simulink model "LoFT_Example3"  (R2024b)
settings: Solver=ode4  StartTime=0.0  StopTime=300  FixedStep=simu.dt  RelTol=1e-3
undefined symbols (not defined in the file): body, circtime, Communication, D1, Delta, irkb, line, LoFT, p0, Pn, s, simu, trip_time, Turbwind, waves, wind
libraries: simulink x350, spsThreePhaseVIMeasurementLib x41, spsThreePhasePISectionLineLib x34, spsThreePhaseParallelRLCLoadLib x21, spsThreePhaseTransformerTwoWindingsLib x14, spsLoadFlowBusLib x10, spsThreePhaseDynamicLoadLib x9, spsSynchronousMachinepuStandardLib x7, spsExcitationSystemLib x7, spsSteamTurbineandGovernorLib x7, spsGenericPowerSystemStabilizerLib x7, spsMultiBandPowerSystemStabilizerLib x7
(part 47 of 49)

== system LoFT_Example3/FOWT System/Subsystem5/FOWT10/Aerodynamics and Local Control Systems/Local Control Systems/Subsystem1/Gain Scheduling ==
  In1 : Inport
  In3 : Inport  Port=2
  In2 : Inport  Port=3
  1-D Lookup Table1 : Lookup_n-D  NumberOfTableDimensions=1  BreakpointsForDimension1=Controller.R.PC_GS_angles  Table=Controller.R.PC_GS_KI  InternalRulePriority=Speed  RndMeth=Simplest
  1-D Lookup Table2 : Lookup_n-D  NumberOfTableDimensions=1  BreakpointsForDimension1=Controller.R.PC_GS_angles  Table=Controller.R.PC_GS_KP  InternalRulePriority=Speed  RndMeth=Simplest
  Add : Sum
  Add1 : Sum
  Constant1 : Constant  Value=90*pi/180
  Delay : Delay  DelayLength=1  InitialCondition=0
  Gain : Gain  Gain=simu.dt
  Product : Product
  Product1 : Product
  Saturation Dynamic : simulink/Discontinuities/Saturation Dynamic  OutMin=[]  OutMax=[]  OutDataTypeStr=Inherit: Same as second input  OutDataType=fixdt(1, 16)  OutScaling=2^-10  DoSatur=off
  Saturation1 : Saturate  UpperLimit=Controller.R.PC_GS_KI(end)  LowerLimit=Controller.R.PC_GS_KI(1)
  Saturation3 : Saturate  UpperLimit=Controller.R.PC_GS_KP(end)  LowerLimit=Controller.R.PC_GS_KP(1)
  Out1 : Outport
  wires:
  1-D Lookup Table1/1 -> Saturation1/1
  1-D Lookup Table2/1 -> Saturation3/1
  In2/1 -> 1-D Lookup Table1/1, 1-D Lookup Table2/1
  In1/1 -> Product/1, Product1/1
  Saturation3/1 -> Product/2
  Saturation1/1 -> Product1/2
  Product1/1 -> Gain/1
  Gain/1 -> Add/1
  Add/1 -> Saturation Dynamic/2
  In3/1 -> Saturation Dynamic/3
  Constant1/1 -> Saturation Dynamic/1
  Saturation Dynamic/1 -> Add1/2, Delay/1
  Delay/1 -> Add/2
  Add1/1 -> Out1/1
  Product/1 -> Add1/1

== system LoFT_Example3/FOWT System/Subsystem5/FOWT2/Aerodynamics and Local Control Systems/Local Control Systems/Subsystem1/Gain Scheduling ==
  In1 : Inport
  In3 : Inport  Port=2
  In2 : Inport  Port=3
  1-D Lookup Table1 : Lookup_n-D  NumberOfTableDimensions=1  BreakpointsForDimension1=Controller.R.PC_GS_angles  Table=Controller.R.PC_GS_KI  InternalRulePriority=Speed  RndMeth=Simplest
  1-D Lookup Table2 : Lookup_n-D  NumberOfTableDimensions=1  BreakpointsForDimension1=Controller.R.PC_GS_angles  Table=Controller.R.PC_GS_KP  InternalRulePriority=Speed  RndMeth=Simplest
  Add : Sum
  Add1 : Sum
  Constant1 : Constant  Value=90*pi/180
  Delay : Delay  DelayLength=1  InitialCondition=0
  Gain : Gain  Gain=simu.dt
  Product : Product
  Product1 : Product
  Saturation Dynamic : simulink/Discontinuities/Saturation Dynamic  OutMin=[]  OutMax=[]  OutDataTypeStr=Inherit: Same as second input  OutDataType=fixdt(1, 16)  OutScaling=2^-10  DoSatur=off
  Saturation1 : Saturate  UpperLimit=Controller.R.PC_GS_KI(end)  LowerLimit=Controller.R.PC_GS_KI(1)
  Saturation3 : Saturate  UpperLimit=Controller.R.PC_GS_KP(end)  LowerLimit=Controller.R.PC_GS_KP(1)
  Out1 : Outport
  wires:
  1-D Lookup Table1/1 -> Saturation1/1
  1-D Lookup Table2/1 -> Saturation3/1
  In2/1 -> 1-D Lookup Table1/1, 1-D Lookup Table2/1
  In1/1 -> Product/1, Product1/1
  Saturation3/1 -> Product/2
  Saturation1/1 -> Product1/2
  Product1/1 -> Gain/1
  Gain/1 -> Add/1
  Add/1 -> Saturation Dynamic/2
  In3/1 -> Saturation Dynamic/3
  Constant1/1 -> Saturation Dynamic/1
  Saturation Dynamic/1 -> Add1/2, Delay/1
  Delay/1 -> Add/2
  Add1/1 -> Out1/1
  Product/1 -> Add1/1

== system LoFT_Example3/FOWT System/Subsystem5/FOWT3/Aerodynamics and Local Control Systems/Local Control Systems/Subsystem1/Gain Scheduling ==
  In1 : Inport
  In3 : Inport  Port=2
  In2 : Inport  Port=3
  1-D Lookup Table1 : Lookup_n-D  NumberOfTableDimensions=1  BreakpointsForDimension1=Controller.R.PC_GS_angles  Table=Controller.R.PC_GS_KI  InternalRulePriority=Speed  RndMeth=Simplest
  1-D Lookup Table2 : Lookup_n-D  NumberOfTableDimensions=1  BreakpointsForDimension1=Controller.R.PC_GS_angles  Table=Controller.R.PC_GS_KP  InternalRulePriority=Speed  RndMeth=Simplest
  Add : Sum
  Add1 : Sum
  Constant1 : Constant  Value=90*pi/180
  Delay : Delay  DelayLength=1  InitialCondition=0
  Gain : Gain  Gain=simu.dt
  Product : Product
  Product1 : Product
  Saturation Dynamic : simulink/Discontinuities/Saturation Dynamic  OutMin=[]  OutMax=[]  OutDataTypeStr=Inherit: Same as second input  OutDataType=fixdt(1, 16)  OutScaling=2^-10  DoSatur=off
  Saturation1 : Saturate  UpperLimit=Controller.R.PC_GS_KI(end)  LowerLimit=Controller.R.PC_GS_KI(1)
  Saturation3 : Saturate  UpperLimit=Controller.R.PC_GS_KP(end)  LowerLimit=Controller.R.PC_GS_KP(1)
  Out1 : Outport
  wires:
  Product/1 -> Add1/1
  Add1/1 -> Out1/1
  Delay/1 -> Add/2
  Saturation Dynamic/1 -> Delay/1, Add1/2
  Constant1/1 -> Saturation Dynamic/1
  In3/1 -> Saturation Dynamic/3
  Add/1 -> Saturation Dynamic/2
  Gain/1 -> Add/1
  Product1/1 -> Gain/1
  Saturation1/1 -> Product1/2
  Saturation3/1 -> Product/2
  In1/1 -> Product1/1, Product/1
  In2/1 -> 1-D Lookup Table2/1, 1-D Lookup Table1/1
  1-D Lookup Table2/1 -> Saturation3/1
  1-D Lookup Table1/1 -> Saturation1/1

== system LoFT_Example3/FOWT System/Subsystem5/FOWT4/Aerodynamics and Local Control Systems/Local Control Systems/Subsystem1/Gain Scheduling ==
  In1 : Inport
  In3 : Inport  Port=2
  In2 : Inport  Port=3
  1-D Lookup Table1 : Lookup_n-D  NumberOfTableDimensions=1  BreakpointsForDimension1=Controller.R.PC_GS_angles  Table=Controller.R.PC_GS_KI  InternalRulePriority=Speed  RndMeth=Simplest
  1-D Lookup Table2 : Lookup_n-D  NumberOfTableDimensions=1  BreakpointsForDimension1=Controller.R.PC_GS_angles  Table=Controller.R.PC_GS_KP  InternalRulePriority=Speed  RndMeth=Simplest
  Add : Sum
  Add1 : Sum
  Constant1 : Constant  Value=90*pi/180
  Delay : Delay  DelayLength=1  InitialCondition=0
  Gain : Gain  Gain=simu.dt
  Product : Product
  Product1 : Product
  Saturation Dynamic : simulink/Discontinuities/Saturation Dynamic  OutMin=[]  OutMax=[]  OutDataTypeStr=Inherit: Same as second input  OutDataType=fixdt(1, 16)  OutScaling=2^-10  DoSatur=off
  Saturation1 : Saturate  UpperLimit=Controller.R.PC_GS_KI(end)  LowerLimit=Controller.R.PC_GS_KI(1)
  Saturation3 : Saturate  UpperLimit=Controller.R.PC_GS_KP(end)  LowerLimit=Controller.R.PC_GS_KP(1)
  Out1 : Outport
  wires:
  1-D Lookup Table1/1 -> Saturation1/1
  1-D Lookup Table2/1 -> Saturation3/1
  In2/1 -> 1-D Lookup Table1/1, 1-D Lookup Table2/1
  In1/1 -> Product/1, Product1/1
  Saturation3/1 -> Product/2
  Saturation1/1 -> Product1/2
  Product1/1 -> Gain/1
  Gain/1 -> Add/1
  Add/1 -> Saturation Dynamic/2
  In3/1 -> Saturation Dynamic/3
  Constant1/1 -> Saturation Dynamic/1
  Saturation Dynamic/1 -> Add1/2, Delay/1
  Delay/1 -> Add/2
  Add1/1 -> Out1/1
  Product/1 -> Add1/1

== system LoFT_Example3/FOWT System/Subsystem5/FOWT5/Aerodynamics and Local Control Systems/Local Control Systems/Subsystem1/Gain Scheduling ==
  In1 : Inport
  In3 : Inport  Port=2
  In2 : Inport  Port=3
  1-D Lookup Table1 : Lookup_n-D  NumberOfTableDimensions=1  BreakpointsForDimension1=Controller.R.PC_GS_angles  Table=Controller.R.PC_GS_KI  InternalRulePriority=Speed  RndMeth=Simplest
  1-D Lookup Table2 : Lookup_n-D  NumberOfTableDimensions=1  BreakpointsForDimension1=Controller.R.PC_GS_angles  Table=Controller.R.PC_GS_KP  InternalRulePriority=Speed  RndMeth=Simplest
  Add : Sum
  Add1 : Sum
  Constant1 : Constant  Value=90*pi/180
  Delay : Delay  DelayLength=1  InitialCondition=0
  Gain : Gain  Gain=simu.dt
  Product : Product
  Product1 : Product
  Saturation Dynamic : simulink/Discontinuities/Saturation Dynamic  OutMin=[]  OutMax=[]  OutDataTypeStr=Inherit: Same as second input  OutDataType=fixdt(1, 16)  OutScaling=2^-10  DoSatur=off
  Saturation1 : Saturate  UpperLimit=Controller.R.PC_GS_KI(end)  LowerLimit=Controller.R.PC_GS_KI(1)
  Saturation3 : Saturate  UpperLimit=Controller.R.PC_GS_KP(end)  LowerLimit=Controller.R.PC_GS_KP(1)
  Out1 : Outport
  wires:
  Product/1 -> Add1/1
  Add1/1 -> Out1/1
  Delay/1 -> Add/2
  Saturation Dynamic/1 -> Delay/1, Add1/2
  Constant1/1 -> Saturation Dynamic/1
  In3/1 -> Saturation Dynamic/3
  Add/1 -> Saturation Dynamic/2
  Gain/1 -> Add/1
  Product1/1 -> Gain/1
  Saturation1/1 -> Product1/2
  Saturation3/1 -> Product/2
  In1/1 -> Product1/1, Product/1
  In2/1 -> 1-D Lookup Table2/1, 1-D Lookup Table1/1
  1-D Lookup Table2/1 -> Saturation3/1
  1-D Lookup Table1/1 -> Saturation1/1

== system LoFT_Example3/FOWT System/Subsystem5/FOWT6/Aerodynamics and Local Control Systems/Local Control Systems/Subsystem1/Gain Scheduling ==
  In1 : Inport
  In3 : Inport  Port=2
  In2 : Inport  Port=3
  1-D Lookup Table1 : Lookup_n-D  NumberOfTableDimensions=1  BreakpointsForDimension1=Controller.R.PC_GS_angles  Table=Controller.R.PC_GS_KI  InternalRulePriority=Speed  RndMeth=Simplest
  1-D Lookup Table2 : Lookup_n-D  NumberOfTableDimensions=1  BreakpointsForDimension1=Controller.R.PC_GS_angles  Table=Controller.R.PC_GS_KP  InternalRulePriority=Speed  RndMeth=Simplest
  Add : Sum
  Add1 : Sum
  Constant1 : Constant  Value=90*pi/180
  Delay : Delay  DelayLength=1  InitialCondition=0
  Gain : Gain  Gain=simu.dt
  Product : Product
  Product1 : Product
  Saturation Dynamic : simulink/Discontinuities/Saturation Dynamic  OutMin=[]  OutMax=[]  OutDataTypeStr=Inherit: Same as second input  OutDataType=fixdt(1, 16)  OutScaling=2^-10  DoSatur=off
  Saturation1 : Saturate  UpperLimit=Controller.R.PC_GS_KI(end)  LowerLimit=Controller.R.PC_GS_KI(1)
  Saturation3 : Saturate  UpperLimit=Controller.R.PC_GS_KP(end)  LowerLimit=Controller.R.PC_GS_KP(1)
  Out1 : Outport
  wires:
  1-D Lookup Table1/1 -> Saturation1/1
  1-D Lookup Table2/1 -> Saturation3/1
  In2/1 -> 1-D Lookup Table1/1, 1-D Lookup Table2/1
  In1/1 -> Product/1, Product1/1
  Saturation3/1 -> Product/2
  Saturation1/1 -> Product1/2
  Product1/1 -> Gain/1
  Gain/1 -> Add/1
  Add/1 -> Saturation Dynamic/2
  In3/1 -> Saturation Dynamic/3
  Constant1/1 -> Saturation Dynamic/1
  Saturation Dynamic/1 -> Add1/2, Delay/1
  Delay/1 -> Add/2
  Add1/1 -> Out1/1
  Product/1 -> Add1/1

== system LoFT_Example3/FOWT System/Subsystem5/FOWT7/Aerodynamics and Local Control Systems/Local Control Systems/Subsystem1/Gain Scheduling ==
  In1 : Inport
  In3 : Inport  Port=2
  In2 : Inport  Port=3
  1-D Lookup Table1 : Lookup_n-D  NumberOfTableDimensions=1  BreakpointsForDimension1=Controller.R.PC_GS_angles  Table=Controller.R.PC_GS_KI  InternalRulePriority=Speed  RndMeth=Simplest
  1-D Lookup Table2 : Lookup_n-D  NumberOfTableDimensions=1  BreakpointsForDimension1=Controller.R.PC_GS_angles  Table=Controller.R.PC_GS_KP  InternalRulePriority=Speed  RndMeth=Simplest
  Add : Sum
  Add1 : Sum
  Constant1 : Constant  Value=90*pi/180
  Delay : Delay  DelayLength=1  InitialCondition=0
  Gain : Gain  Gain=simu.dt
  Product : Product
  Product1 : Product
  Saturation Dynamic : simulink/Discontinuities/Saturation Dynamic  OutMin=[]  OutMax=[]  OutDataTypeStr=Inherit: Same as second input  OutDataType=fixdt(1, 16)  OutScaling=2^-10  DoSatur=off
  Saturation1 : Saturate  UpperLimit=Controller.R.PC_GS_KI(end)  LowerLimit=Controller.R.PC_GS_KI(1)
  Saturation3 : Saturate  UpperLimit=Controller.R.PC_GS_KP(end)  LowerLimit=Controller.R.PC_GS_KP(1)
  Out1 : Outport
  wires:
  Product/1 -> Add1/1
  Add1/1 -> Out1/1
  Delay/1 -> Add/2
  Saturation Dynamic/1 -> Delay/1, Add1/2
  Constant1/1 -> Saturation Dynamic/1
  In3/1 -> Saturation Dynamic/3
  Add/1 -> Saturation Dynamic/2
  Gain/1 -> Add/1
  Product1/1 -> Gain/1
  Saturation1/1 -> Product1/2
  Saturation3/1 -> Product/2
  In1/1 -> Product1/1, Product/1
  In2/1 -> 1-D Lookup Table2/1, 1-D Lookup Table1/1
  1-D Lookup Table2/1 -> Saturation3/1
  1-D Lookup Table1/1 -> Saturation1/1

== system LoFT_Example3/FOWT System/Subsystem5/FOWT8/Aerodynamics and Local Control Systems/Local Control Systems/Subsystem1/Gain Scheduling ==
  In1 : Inport
  In3 : Inport  Port=2
  In2 : Inport  Port=3
  1-D Lookup Table1 : Lookup_n-D  NumberOfTableDimensions=1  BreakpointsForDimension1=Controller.R.PC_GS_angles  Table=Controller.R.PC_GS_KI  InternalRulePriority=Speed  RndMeth=Simplest
  1-D Lookup Table2 : Lookup_n-D  NumberOfTableDimensions=1  BreakpointsForDimension1=Controller.R.PC_GS_angles  Table=Controller.R.PC_GS_KP  InternalRulePriority=Speed  RndMeth=Simplest
  Add : Sum
  Add1 : Sum
  Constant1 : Constant  Value=90*pi/180
  Delay : Delay  DelayLength=1  InitialCondition=0
  Gain : Gain  Gain=simu.dt
  Product : Product
  Product1 : Product
  Saturation Dynamic : simulink/Discontinuities/Saturation Dynamic  OutMin=[]  OutMax=[]  OutDataTypeStr=Inherit: Same as second input  OutDataType=fixdt(1, 16)  OutScaling=2^-10  DoSatur=off
  Saturation1 : Saturate  UpperLimit=Controller.R.PC_GS_KI(end)  LowerLimit=Controller.R.PC_GS_KI(1)
  Saturation3 : Saturate  UpperLimit=Controller.R.PC_GS_KP(end)  LowerLimit=Controller.R.PC_GS_KP(1)
  Out1 : Outport
  wires:
  1-D Lookup Table1/1 -> Saturation1/1
  1-D Lookup Table2/1 -> Saturation3/1
  In2/1 -> 1-D Lookup Table1/1, 1-D Lookup Table2/1
  In1/1 -> Product/1, Product1/1
  Saturation3/1 -> Product/2
  Saturation1/1 -> Product1/2
  Product1/1 -> Gain/1
  Gain/1 -> Add/1
  Add/1 -> Saturation Dynamic/2
  In3/1 -> Saturation Dynamic/3
  Constant1/1 -> Saturation Dynamic/1
  Saturation Dynamic/1 -> Add1/2, Delay/1
  Delay/1 -> Add/2
  Add1/1 -> Out1/1
  Product/1 -> Add1/1

== system LoFT_Example3/FOWT System/Subsystem5/FOWT9/Aerodynamics and Local Control Systems/Local Control Systems/Subsystem1/Gain Scheduling ==
  In1 : Inport
  In3 : Inport  Port=2
  In2 : Inport  Port=3
  1-D Lookup Table1 : Lookup_n-D  NumberOfTableDimensions=1  BreakpointsForDimension1=Controller.R.PC_GS_angles  Table=Controller.R.PC_GS_KI  InternalRulePriority=Speed  RndMeth=Simplest
  1-D Lookup Table2 : Lookup_n-D  NumberOfTableDimensions=1  BreakpointsForDimension1=Controller.R.PC_GS_angles  Table=Controller.R.PC_GS_KP  InternalRulePriority=Speed  RndMeth=Simplest
  Add : Sum
  Add1 : Sum
  Constant1 : Constant  Value=90*pi/180
  Delay : Delay  DelayLength=1  InitialCondition=0
  Gain : Gain  Gain=simu.dt
  Product : Product
  Product1 : Product
  Saturation Dynamic : simulink/Discontinuities/Saturation Dynamic  OutMin=[]  OutMax=[]  OutDataTypeStr=Inherit: Same as second input  OutDataType=fixdt(1, 16)  OutScaling=2^-10  DoSatur=off
  Saturation1 : Saturate  UpperLimit=Controller.R.PC_GS_KI(end)  LowerLimit=Controller.R.PC_GS_KI(1)
  Saturation3 : Saturate  UpperLimit=Controller.R.PC_GS_KP(end)  LowerLimit=Controller.R.PC_GS_KP(1)
  Out1 : Outport
  wires:
  Product/1 -> Add1/1
  Add1/1 -> Out1/1
  Delay/1 -> Add/2
  Saturation Dynamic/1 -> Delay/1, Add1/2
  Constant1/1 -> Saturation Dynamic/1
  In3/1 -> Saturation Dynamic/3
  Add/1 -> Saturation Dynamic/2
  Gain/1 -> Add/1
  Product1/1 -> Gain/1
  Saturation1/1 -> Product1/2
  Saturation3/1 -> Product/2
  In1/1 -> Product1/1, Product/1
  In2/1 -> 1-D Lookup Table2/1, 1-D Lookup Table1/1
  1-D Lookup Table2/1 -> Saturation3/1
  1-D Lookup Table1/1 -> Saturation1/1

== system LoFT_Example3/FOWT System/Subsystem7/FOWT1/Aerodynamics and Local Control Systems/Local Control Systems/Subsystem1/Gain Scheduling ==
  In1 : Inport
  In3 : Inport  Port=2
  In2 : Inport  Port=3
  1-D Lookup Table1 : Lookup_n-D  NumberOfTableDimensions=1  BreakpointsForDimension1=Controller.R.PC_GS_angles  Table=Controller.R.PC_GS_KI  InternalRulePriority=Speed  RndMeth=Simplest
  1-D Lookup Table2 : Lookup_n-D  NumberOfTableDimensions=1  BreakpointsForDimension1=Controller.R.PC_GS_angles  Table=Controller.R.PC_GS_KP  InternalRulePriority=Speed  RndMeth=Simplest
  Add : Sum
  Add1 : Sum
  Constant1 : Constant  Value=90*pi/180
  Delay : Delay  DelayLength=1  InitialCondition=0
  Gain : Gain  Gain=simu.dt
  Product : Product
  Product1 : Product
  Saturation Dynamic : simulink/Discontinuities/Saturation Dynamic  OutMin=[]  OutMax=[]  OutDataTypeStr=Inherit: Same as second input  OutDataType=fixdt(1, 16)  OutScaling=2^-10  DoSatur=off
  Saturation1 : Saturate  UpperLimit=Controller.R.PC_GS_KI(end)  LowerLimit=Controller.R.PC_GS_KI(1)
  Saturation3 : Saturate  UpperLimit=Controller.R.PC_GS_KP(end)  LowerLimit=Controller.R.PC_GS_KP(1)
  Out1 : Outport
  wires:
  1-D Lookup Table1/1 -> Saturation1/1
  1-D Lookup Table2/1 -> Saturation3/1
  In2/1 -> 1-D Lookup Table1/1, 1-D Lookup Table2/1
  In1/1 -> Product/1, Product1/1
  Saturation3/1 -> Product/2
  Saturation1/1 -> Product1/2
  Product1/1 -> Gain/1
  Gain/1 -> Add/1
  Add/1 -> Saturation Dynamic/2
  In3/1 -> Saturation Dynamic/3
  Constant1/1 -> Saturation Dynamic/1
  Saturation Dynamic/1 -> Add1/2, Delay/1
  Delay/1 -> Add/2
  Add1/1 -> Out1/1
  Product/1 -> Add1/1

== system LoFT_Example3/FOWT System/Subsystem7/FOWT10/Aerodynamics and Local Control Systems/Local Control Systems/Subsystem1/Gain Scheduling ==
  In1 : Inport
  In3 : Inport  Port=2
  In2 : Inport  Port=3
  1-D Lookup Table1 : Lookup_n-D  NumberOfTableDimensions=1  BreakpointsForDimension1=Controller.R.PC_GS_angles  Table=Controller.R.PC_GS_KI  InternalRulePriority=Speed  RndMeth=Simplest
  1-D Lookup Table2 : Lookup_n-D  NumberOfTableDimensions=1  BreakpointsForDimension1=Controller.R.PC_GS_angles  Table=Controller.R.PC_GS_KP  InternalRulePriority=Speed  RndMeth=Simplest
  Add : Sum
  Add1 : Sum
  Constant1 : Constant  Value=90*pi/180
  Delay : Delay  DelayLength=1  InitialCondition=0
  Gain : Gain  Gain=simu.dt
  Product : Product
  Product1 : Product
  Saturation Dynamic : simulink/Discontinuities/Saturation Dynamic  OutMin=[]  OutMax=[]  OutDataTypeStr=Inherit: Same as second input  OutDataType=fixdt(1, 16)  OutScaling=2^-10  DoSatur=off
  Saturation1 : Saturate  UpperLimit=Controller.R.PC_GS_KI(end)  LowerLimit=Controller.R.PC_GS_KI(1)
  Saturation3 : Saturate  UpperLimit=Controller.R.PC_GS_KP(end)  LowerLimit=Controller.R.PC_GS_KP(1)
  Out1 : Outport
  wires:
  Product/1 -> Add1/1
  Add1/1 -> Out1/1
  Delay/1 -> Add/2
  Saturation Dynamic/1 -> Delay/1, Add1/2
  Constant1/1 -> Saturation Dynamic/1
  In3/1 -> Saturation Dynamic/3
  Add/1 -> Saturation Dynamic/2
  Gain/1 -> Add/1
  Product1/1 -> Gain/1
  Saturation1/1 -> Product1/2
  Saturation3/1 -> Product/2
  In1/1 -> Product1/1, Product/1
  In2/1 -> 1-D Lookup Table2/1, 1-D Lookup Table1/1
  1-D Lookup Table2/1 -> Saturation3/1
  1-D Lookup Table1/1 -> Saturation1/1

== system LoFT_Example3/FOWT System/Subsystem7/FOWT2/Aerodynamics and Local Control Systems/Local Control Systems/Subsystem1/Gain Scheduling ==
  In1 : Inport
  In3 : Inport  Port=2
  In2 : Inport  Port=3
  1-D Lookup Table1 : Lookup_n-D  NumberOfTableDimensions=1  BreakpointsForDimension1=Controller.R.PC_GS_angles  Table=Controller.R.PC_GS_KI  InternalRulePriority=Speed  RndMeth=Simplest
  1-D Lookup Table2 : Lookup_n-D  NumberOfTableDimensions=1  BreakpointsForDimension1=Controller.R.PC_GS_angles  Table=Controller.R.PC_GS_KP  InternalRulePriority=Speed  RndMeth=Simplest
  Add : Sum
  Add1 : Sum
  Constant1 : Constant  Value=90*pi/180
  Delay : Delay  DelayLength=1  InitialCondition=0
  Gain : Gain  Gain=simu.dt
  Product : Product
  Product1 : Product
  Saturation Dynamic : simulink/Discontinuities/Saturation Dynamic  OutMin=[]  OutMax=[]  OutDataTypeStr=Inherit: Same as second input  OutDataType=fixdt(1, 16)  OutScaling=2^-10  DoSatur=off
  Saturation1 : Saturate  UpperLimit=Controller.R.PC_GS_KI(end)  LowerLimit=Controller.R.PC_GS_KI(1)
  Saturation3 : Saturate  UpperLimit=Controller.R.PC_GS_KP(end)  LowerLimit=Controller.R.PC_GS_KP(1)
  Out1 : Outport
  wires:
  Product/1 -> Add1/1
  Add1/1 -> Out1/1
  Delay/1 -> Add/2
  Saturation Dynamic/1 -> Delay/1, Add1/2
  Constant1/1 -> Saturation Dynamic/1
  In3/1 -> Saturation Dynamic/3
  Add/1 -> Saturation Dynamic/2
  Gain/1 -> Add/1
  Product1/1 -> Gain/1
  Saturation1/1 -> Product1/2
  Saturation3/1 -> Product/2
  In1/1 -> Product1/1, Product/1
  In2/1 -> 1-D Lookup Table2/1, 1-D Lookup Table1/1
  1-D Lookup Table2/1 -> Saturation3/1
  1-D Lookup Table1/1 -> Saturation1/1

== system LoFT_Example3/FOWT System/Subsystem7/FOWT3/Aerodynamics and Local Control Systems/Local Control Systems/Subsystem1/Gain Scheduling ==
  In1 : Inport
  In3 : Inport  Port=2
  In2 : Inport  Port=3
  1-D Lookup Table1 : Lookup_n-D  NumberOfTableDimensions=1  BreakpointsForDimension1=Controller.R.PC_GS_angles  Table=Controller.R.PC_GS_KI  InternalRulePriority=Speed  RndMeth=Simplest
  1-D Lookup Table2 : Lookup_n-D  NumberOfTableDimensions=1  BreakpointsForDimension1=Controller.R.PC_GS_angles  Table=Controller.R.PC_GS_KP  InternalRulePriority=Speed  RndMeth=Simplest
  Add : Sum
  Add1 : Sum
  Constant1 : Constant  Value=90*pi/180
  Delay : Delay  DelayLength=1  InitialCondition=0
  Gain : Gain  Gain=simu.dt
  Product : Product
  Product1 : Product
  Saturation Dynamic : simulink/Discontinuities/Saturation Dynamic  OutMin=[]  OutMax=[]  OutDataTypeStr=Inherit: Same as second input  OutDataType=fixdt(1, 16)  OutScaling=2^-10  DoSatur=off
  Saturation1 : Saturate  UpperLimit=Controller.R.PC_GS_KI(end)  LowerLimit=Controller.R.PC_GS_KI(1)
  Saturation3 : Saturate  UpperLimit=Controller.R.PC_GS_KP(end)  LowerLimit=Controller.R.PC_GS_KP(1)
  Out1 : Outport
  wires:
  1-D Lookup Table1/1 -> Saturation1/1
  1-D Lookup Table2/1 -> Saturation3/1
  In2/1 -> 1-D Lookup Table1/1, 1-D Lookup Table2/1
  In1/1 -> Product/1, Product1/1
  Saturation3/1 -> Product/2
  Saturation1/1 -> Product1/2
  Product1/1 -> Gain/1
  Gain/1 -> Add/1
  Add/1 -> Saturation Dynamic/2
  In3/1 -> Saturation Dynamic/3
  Constant1/1 -> Saturation Dynamic/1
  Saturation Dynamic/1 -> Add1/2, Delay/1
  Delay/1 -> Add/2
  Add1/1 -> Out1/1
  Product/1 -> Add1/1

== system LoFT_Example3/FOWT System/Subsystem7/FOWT4/Aerodynamics and Local Control Systems/Local Control Systems/Subsystem1/Gain Scheduling ==
  In1 : Inport
  In3 : Inport  Port=2
  In2 : Inport  Port=3
  1-D Lookup Table1 : Lookup_n-D  NumberOfTableDimensions=1  BreakpointsForDimension1=Controller.R.PC_GS_angles  Table=Controller.R.PC_GS_KI  InternalRulePriority=Speed  RndMeth=Simplest
  1-D Lookup Table2 : Lookup_n-D  NumberOfTableDimensions=1  BreakpointsForDimension1=Controller.R.PC_GS_angles  Table=Controller.R.PC_GS_KP  InternalRulePriority=Speed  RndMeth=Simplest
  Add : Sum
  Add1 : Sum
  Constant1 : Constant  Value=90*pi/180
  Delay : Delay  DelayLength=1  InitialCondition=0
  Gain : Gain  Gain=simu.dt
  Product : Product
  Product1 : Product
  Saturation Dynamic : simulink/Discontinuities/Saturation Dynamic  OutMin=[]  OutMax=[]  OutDataTypeStr=Inherit: Same as second input  OutDataType=fixdt(1, 16)  OutScaling=2^-10  DoSatur=off
  Saturation1 : Saturate  UpperLimit=Controller.R.PC_GS_KI(end)  LowerLimit=Controller.R.PC_GS_KI(1)
  Saturation3 : Saturate  UpperLimit=Controller.R.PC_GS_KP(end)  LowerLimit=Controller.R.PC_GS_KP(1)
  Out1 : Outport
  wires:
  Product/1 -> Add1/1
  Add1/1 -> Out1/1
  Delay/1 -> Add/2
  Saturation Dynamic/1 -> Delay/1, Add1/2
  Constant1/1 -> Saturation Dynamic/1
  In3/1 -> Saturation Dynamic/3
  Add/1 -> Saturation Dynamic/2
  Gain/1 -> Add/1
  Product1/1 -> Gain/1
  Saturation1/1 -> Product1/2
  Saturation3/1 -> Product/2
  In1/1 -> Product1/1, Product/1
  In2/1 -> 1-D Lookup Table2/1, 1-D Lookup Table1/1
  1-D Lookup Table2/1 -> Saturation3/1
  1-D Lookup Table1/1 -> Saturation1/1

== system LoFT_Example3/FOWT System/Subsystem7/FOWT5/Aerodynamics and Local Control Systems/Local Control Systems/Subsystem1/Gain Scheduling ==
  In1 : Inport
  In3 : Inport  Port=2
  In2 : Inport  Port=3
  1-D Lookup Table1 : Lookup_n-D  NumberOfTableDimensions=1  BreakpointsForDimension1=Controller.R.PC_GS_angles  Table=Controller.R.PC_GS_KI  InternalRulePriority=Speed  RndMeth=Simplest
  1-D Lookup Table2 : Lookup_n-D  NumberOfTableDimensions=1  BreakpointsForDimension1=Controller.R.PC_GS_angles  Table=Controller.R.PC_GS_KP  InternalRulePriority=Speed  RndMeth=Simplest
  Add : Sum
  Add1 : Sum
  Constant1 : Constant  Value=90*pi/180
  Delay : Delay  DelayLength=1  InitialCondition=0
  Gain : Gain  Gain=simu.dt
  Product : Product
  Product1 : Product
  Saturation Dynamic : simulink/Discontinuities/Saturation Dynamic  OutMin=[]  OutMax=[]  OutDataTypeStr=Inherit: Same as second input  OutDataType=fixdt(1, 16)  OutScaling=2^-10  DoSatur=off
  Saturation1 : Saturate  UpperLimit=Controller.R.PC_GS_KI(end)  LowerLimit=Controller.R.PC_GS_KI(1)
  Saturation3 : Saturate  UpperLimit=Controller.R.PC_GS_KP(end)  LowerLimit=Controller.R.PC_GS_KP(1)
  Out1 : Outport
  wires:
  1-D Lookup Table1/1 -> Saturation1/1
  1-D Lookup Table2/1 -> Saturation3/1
  In2/1 -> 1-D Lookup Table1/1, 1-D Lookup Table2/1
  In1/1 -> Product/1, Product1/1
  Saturation3/1 -> Product/2
  Saturation1/1 -> Product1/2
  Product1/1 -> Gain/1
  Gain/1 -> Add/1
  Add/1 -> Saturation Dynamic/2
  In3/1 -> Saturation Dynamic/3
  Constant1/1 -> Saturation Dynamic/1
  Saturation Dynamic/1 -> Add1/2, Delay/1
  Delay/1 -> Add/2
  Add1/1 -> Out1/1
  Product/1 -> Add1/1

== system LoFT_Example3/FOWT System/Subsystem7/FOWT6/Aerodynamics and Local Control Systems/Local Control Systems/Subsystem1/Gain Scheduling ==
  In1 : Inport
  In3 : Inport  Port=2
  In2 : Inport  Port=3
  1-D Lookup Table1 : Lookup_n-D  NumberOfTableDimensions=1  BreakpointsForDimension1=Controller.R.PC_GS_angles  Table=Controller.R.PC_GS_KI  InternalRulePriority=Speed  RndMeth=Simplest
  1-D Lookup Table2 : Lookup_n-D  NumberOfTableDimensions=1  BreakpointsForDimension1=Controller.R.PC_GS_angles  Table=Controller.R.PC_GS_KP  InternalRulePriority=Speed  RndMeth=Simplest
  Add : Sum
  Add1 : Sum
  Constant1 : Constant  Value=90*pi/180
  Delay : Delay  DelayLength=1  InitialCondition=0
  Gain : Gain  Gain=simu.dt
  Product : Product
  Product1 : Product
  Saturation Dynamic : simulink/Discontinuities/Saturation Dynamic  OutMin=[]  OutMax=[]  OutDataTypeStr=Inherit: Same as second input  OutDataType=fixdt(1, 16)  OutScaling=2^-10  DoSatur=off
  Saturation1 : Saturate  UpperLimit=Controller.R.PC_GS_KI(end)  LowerLimit=Controller.R.PC_GS_KI(1)
  Saturation3 : Saturate  UpperLimit=Controller.R.PC_GS_KP(end)  LowerLimit=Controller.R.PC_GS_KP(1)
  Out1 : Outport
  wires:
  Product/1 -> Add1/1
  Add1/1 -> Out1/1
  Delay/1 -> Add/2
  Saturation Dynamic/1 -> Delay/1, Add1/2
  Constant1/1 -> Saturation Dynamic/1
  In3/1 -> Saturation Dynamic/3
  Add/1 -> Saturation Dynamic/2
  Gain/1 -> Add/1
  Product1/1 -> Gain/1
  Saturation1/1 -> Product1/2
  Saturation3/1 -> Product/2
  In1/1 -> Product1/1, Product/1
  In2/1 -> 1-D Lookup Table2/1, 1-D Lookup Table1/1
  1-D Lookup Table2/1 -> Saturation3/1
  1-D Lookup Table1/1 -> Saturation1/1

== system LoFT_Example3/FOWT System/Subsystem7/FOWT7/Aerodynamics and Local Control Systems/Local Control Systems/Subsystem1/Gain Scheduling ==
  In1 : Inport
  In3 : Inport  Port=2
  In2 : Inport  Port=3
  1-D Lookup Table1 : Lookup_n-D  NumberOfTableDimensions=1  BreakpointsForDimension1=Controller.R.PC_GS_angles  Table=Controller.R.PC_GS_KI  InternalRulePriority=Speed  RndMeth=Simplest
  1-D Lookup Table2 : Lookup_n-D  NumberOfTableDimensions=1  BreakpointsForDimension1=Controller.R.PC_GS_angles  Table=Controller.R.PC_GS_KP  InternalRulePriority=Speed  RndMeth=Simplest
  Add : Sum
  Add1 : Sum
  Constant1 : Constant  Value=90*pi/180
  Delay : Delay  DelayLength=1  InitialCondition=0
  Gain : Gain  Gain=simu.dt
  Product : Product
  Product1 : Product
  Saturation Dynamic : simulink/Discontinuities/Saturation Dynamic  OutMin=[]  OutMax=[]  OutDataTypeStr=Inherit: Same as second input  OutDataType=fixdt(1, 16)  OutScaling=2^-10  DoSatur=off
  Saturation1 : Saturate  UpperLimit=Controller.R.PC_GS_KI(end)  LowerLimit=Controller.R.PC_GS_KI(1)
  Saturation3 : Saturate  UpperLimit=Controller.R.PC_GS_KP(end)  LowerLimit=Controller.R.PC_GS_KP(1)
  Out1 : Outport
  wires:
  1-D Lookup Table1/1 -> Saturation1/1
  1-D Lookup Table2/1 -> Saturation3/1
  In2/1 -> 1-D Lookup Table1/1, 1-D Lookup Table2/1
  In1/1 -> Product/1, Product1/1
  Saturation3/1 -> Product/2
  Saturation1/1 -> Product1/2
  Product1/1 -> Gain/1
  Gain/1 -> Add/1
  Add/1 -> Saturation Dynamic/2
  In3/1 -> Saturation Dynamic/3
  Constant1/1 -> Saturation Dynamic/1
  Saturation Dynamic/1 -> Add1/2, Delay/1
  Delay/1 -> Add/2
  Add1/1 -> Out1/1
  Product/1 -> Add1/1

== system LoFT_Example3/FOWT System/Subsystem7/FOWT8/Aerodynamics and Local Control Systems/Local Control Systems/Subsystem1/Gain Scheduling ==
  In1 : Inport
  In3 : Inport  Port=2
  In2 : Inport  Port=3
  1-D Lookup Table1 : Lookup_n-D  NumberOfTableDimensions=1  BreakpointsForDimension1=Controller.R.PC_GS_angles  Table=Controller.R.PC_GS_KI  InternalRulePriority=Speed  RndMeth=Simplest
  1-D Lookup Table2 : Lookup_n-D  NumberOfTableDimensions=1  BreakpointsForDimension1=Controller.R.PC_GS_angles  Table=Controller.R.PC_GS_KP  InternalRulePriority=Speed  RndMeth=Simplest
  Add : Sum
  Add1 : Sum
  Constant1 : Constant  Value=90*pi/180
  Delay : Delay  DelayLength=1  InitialCondition=0
  Gain : Gain  Gain=simu.dt
  Product : Product
  Product1 : Product
  Saturation Dynamic : simulink/Discontinuities/Saturation Dynamic  OutMin=[]  OutMax=[]  OutDataTypeStr=Inherit: Same as second input  OutDataType=fixdt(1, 16)  OutScaling=2^-10  DoSatur=off
  Saturation1 : Saturate  UpperLimit=Controller.R.PC_GS_KI(end)  LowerLimit=Controller.R.PC_GS_KI(1)
  Saturation3 : Saturate  UpperLimit=Controller.R.PC_GS_KP(end)  LowerLimit=Controller.R.PC_GS_KP(1)
  Out1 : Outport
  wires:
  Product/1 -> Add1/1
  Add1/1 -> Out1/1
  Delay/1 -> Add/2
  Saturation Dynamic/1 -> Delay/1, Add1/2
  Constant1/1 -> Saturation Dynamic/1
  In3/1 -> Saturation Dynamic/3
  Add/1 -> Saturation Dynamic/2
  Gain/1 -> Add/1
  Product1/1 -> Gain/1
  Saturation1/1 -> Product1/2
  Saturation3/1 -> Product/2
  In1/1 -> Product1/1, Product/1
  In2/1 -> 1-D Lookup Table2/1, 1-D Lookup Table1/1
  1-D Lookup Table2/1 -> Saturation3/1
  1-D Lookup Table1/1 -> Saturation1/1

== system LoFT_Example3/FOWT System/Subsystem7/FOWT9/Aerodynamics and Local Control Systems/Local Control Systems/Subsystem1/Gain Scheduling ==
  In1 : Inport
  In3 : Inport  Port=2
  In2 : Inport  Port=3
  1-D Lookup Table1 : Lookup_n-D  NumberOfTableDimensions=1  BreakpointsForDimension1=Controller.R.PC_GS_angles  Table=Controller.R.PC_GS_KI  InternalRulePriority=Speed  RndMeth=Simplest
  1-D Lookup Table2 : Lookup_n-D  NumberOfTableDimensions=1  BreakpointsForDimension1=Controller.R.PC_GS_angles  Table=Controller.R.PC_GS_KP  InternalRulePriority=Speed  RndMeth=Simplest
  Add : Sum
  Add1 : Sum
  Constant1 : Constant  Value=90*pi/180
  Delay : Delay  DelayLength=1  InitialCondition=0
  Gain : Gain  Gain=simu.dt
  Product : Product
  Product1 : Product
  Saturation Dynamic : simulink/Discontinuities/Saturation Dynamic  OutMin=[]  OutMax=[]  OutDataTypeStr=Inherit: Same as second input  OutDataType=fixdt(1, 16)  OutScaling=2^-10  DoSatur=off
  Saturation1 : Saturate  UpperLimit=Controller.R.PC_GS_KI(end)  LowerLimit=Controller.R.PC_GS_KI(1)
  Saturation3 : Saturate  UpperLimit=Controller.R.PC_GS_KP(end)  LowerLimit=Controller.R.PC_GS_KP(1)
  Out1 : Outport
  wires:
  1-D Lookup Table1/1 -> Saturation1/1
  1-D Lookup Table2/1 -> Saturation3/1
  In2/1 -> 1-D Lookup Table1/1, 1-D Lookup Table2/1
  In1/1 -> Product/1, Product1/1
  Saturation3/1 -> Product/2
  Saturation1/1 -> Product1/2
  Product1/1 -> Gain/1
  Gain/1 -> Add/1
  Add/1 -> Saturation Dynamic/2
  In3/1 -> Saturation Dynamic/3
  Constant1/1 -> Saturation Dynamic/1
  Saturation Dynamic/1 -> Add1/2, Delay/1
  Delay/1 -> Add/2
  Add1/1 -> Out1/1
  Product/1 -> Add1/1

== system LoFT_Example3/Onshore grid/Onshore Grid/Subsystem/SG1/Regulators1/Turbine  & Excitation Regulators Mac2/Stabilisateur ==
  Pm : Inport
  Pe : Inport  Port=2
  dw : Inport  Port=3
  Generic Power System Stabilizer : spsGenericPowerSystemStabilizerLib/Generic Power System Stabilizer  Tsensor=15e-3  K=2.5  Twashout=1  Tleadlag1="[0.06  1]"  Tleadlag2="[0  0]"  VSlimits=[-0.15 0.15]  Vinit=0  Plot_On=off  MagdB_On=on  FreqRange=logspace(-2,2,500)
  Ground1 : Ground
  Multi-Band Power System Stabilizer : spsMultiBandPowerSystemStabilizerLib/Multi-Band Power System Stabilizer  OperationMode=Simplified settings  Kg=0.7  GL=[0.2 10]  GI=[0.9 30]  GH=[12.0 115]  GLd=[66 66 9.4]  TcLF=[1.667 2 0 0 0 0 2 2.4 0 0 0 0 1 1]  GId=[66 66 47.6]  TcIF=[1 1 0.25 0.3 0 0 1 1 0.3 0.36 0 0 0 0]  GHd=[66 66 233]  TcHF="[0.01 0.012 0 0 0 0  0.012 0.0144 0 0 0 0 1 1]"  LIM=[.075 .15 .15 .15]  Plot_On=off  MagdB_On=on  FreqRange=logspace(-2,2,500)
  Multiport Switch : MultiPortSwitch
  Sum2 : Sum  Inputs=+-  InputSameDT=on  SaturateOnIntegerOverflow=on  OutDataTypeStr=Inherit: Same as first input
  Stab : Outport  InitialOutput=0  VectorParamsAs1DForOutWhenUnconnected=off
  wires:
  Multi-Band Power System Stabilizer/1 -> Multiport Switch/4
  dw/1 -> Multi-Band Power System Stabilizer/1
  [PSS_select] -> Multiport Switch/1
  Ground1/1 -> Multiport Switch/2
  Pe/1 -> Sum2/2
  Pm/1 -> Sum2/1
  Sum2/1 -> Generic Power System Stabilizer/1
  Generic Power System Stabilizer/1 -> Multiport Switch/3
  Multiport Switch/1 -> Stab/1

== system LoFT_Example3/Onshore grid/Onshore Grid/Subsystem/SG2/Regulators2/Turbine  & Excitation Regulators Mac2/Stabilisateur ==
  Pm : Inport
  Pe : Inport  Port=2
  dw : Inport  Port=3
  Generic Power System Stabilizer : spsGenericPowerSystemStabilizerLib/Generic Power System Stabilizer  Tsensor=15e-3  K=2.5  Twashout=1  Tleadlag1="[0.06  1]"  Tleadlag2="[0  0]"  VSlimits=[-0.15 0.15]  Vinit=0  Plot_On=off  MagdB_On=on  FreqRange=logspace(-2,2,500)
  Ground1 : Ground
  Multi-Band Power System Stabilizer : spsMultiBandPowerSystemStabilizerLib/Multi-Band Power System Stabilizer  OperationMode=Simplified settings  Kg=0.7  GL=[0.2 10]  GI=[0.9 30]  GH=[12.0 115]  GLd=[66 66 9.4]  TcLF=[1.667 2 0 0 0 0 2 2.4 0 0 0 0 1 1]  GId=[66 66 47.6]  TcIF=[1 1 0.25 0.3 0 0 1 1 0.3 0.36 0 0 0 0]  GHd=[66 66 233]  TcHF="[0.01 0.012 0 0 0 0  0.012 0.0144 0 0 0 0 1 1]"  LIM=[.075 .15 .15 .15]  Plot_On=off  MagdB_On=on  FreqRange=logspace(-2,2,500)
  Multiport Switch : MultiPortSwitch
  Sum2 : Sum  Inputs=+-  InputSameDT=on  SaturateOnIntegerOverflow=on  OutDataTypeStr=Inherit: Same as first input
  Stab : Outport  InitialOutput=0  VectorParamsAs1DForOutWhenUnconnected=off
  wires:
  Multi-Band Power System Stabilizer/1 -> Multiport Switch/4
  dw/1 -> Multi-Band Power System Stabilizer/1
  [PSS_select] -> Multiport Switch/1
  Ground1/1 -> Multiport Switch/2
  Pe/1 -> Sum2/2
  Pm/1 -> Sum2/1
  Sum2/1 -> Generic Power System Stabilizer/1
  Generic Power System Stabilizer/1 -> Multiport Switch/3
  Multiport Switch/1 -> Stab/1

== system LoFT_Example3/Onshore grid/Onshore Grid/Subsystem/SG4/Regulators4/Turbine  & Excitation Regulators Mac2/Stabilisateur ==
  Pm : Inport
  Pe : Inport  Port=2
  dw : Inport  Port=3
  Generic Power System Stabilizer : spsGenericPowerSystemStabilizerLib/Generic Power System Stabilizer  Tsensor=15e-3  K=2.5  Twashout=1  Tleadlag1="[0.06  1]"  Tleadlag2="[0  0]"  VSlimits=[-0.15 0.15]  Vinit=0  Plot_On=off  MagdB_On=on  FreqRange=logspace(-2,2,500)
  Ground1 : Ground
  Multi-Band Power System Stabilizer : spsMultiBandPowerSystemStabilizerLib/Multi-Band Power System Stabilizer  OperationMode=Simplified settings  Kg=0.7  GL=[0.2 10]  GI=[0.9 30]  GH=[12.0 115]  GLd=[66 66 9.4]  TcLF=[1.667 2 0 0 0 0 2 2.4 0 0 0 0 1 1]  GId=[66 66 47.6]  TcIF=[1 1 0.25 0.3 0 0 1 1 0.3 0.36 0 0 0 0]  GHd=[66 66 233]  TcHF="[0.01 0.012 0 0 0 0  0.012 0.0144 0 0 0 0 1 1]"  LIM=[.075 .15 .15 .15]  Plot_On=off  MagdB_On=on  FreqRange=logspace(-2,2,500)
  Multiport Switch : MultiPortSwitch
  Sum2 : Sum  Inputs=+-  InputSameDT=on  SaturateOnIntegerOverflow=on  OutDataTypeStr=Inherit: Same as first input
  Stab : Outport  InitialOutput=0  VectorParamsAs1DForOutWhenUnconnected=off
  wires:
  Multi-Band Power System Stabilizer/1 -> Multiport Switch/4
  dw/1 -> Multi-Band Power System Stabilizer/1
  [PSS_select] -> Multiport Switch/1
  Ground1/1 -> Multiport Switch/2
  Pe/1 -> Sum2/2
  Pm/1 -> Sum2/1
  Sum2/1 -> Generic Power System Stabilizer/1
  Generic Power System Stabilizer/1 -> Multiport Switch/3
  Multiport Switch/1 -> Stab/1

== system LoFT_Example3/Onshore grid/Onshore Grid/Subsystem/SG5/Regulators5/Turbine  & Excitation Regulators Mac2/Stabilisateur ==
  Pm : Inport
  Pe : Inport  Port=2
  dw : Inport  Port=3
  Generic Power System Stabilizer : spsGenericPowerSystemStabilizerLib/Generic Power System Stabilizer  Tsensor=15e-3  K=2.5  Twashout=1  Tleadlag1="[0.06  1]"  Tleadlag2="[0  0]"  VSlimits=[-0.15 0.15]  Vinit=0  Plot_On=off  MagdB_On=on  FreqRange=logspace(-2,2,500)
  Ground1 : Ground
  Multi-Band Power System Stabilizer : spsMultiBandPowerSystemStabilizerLib/Multi-Band Power System Stabilizer  OperationMode=Simplified settings  Kg=0.7  GL=[0.2 10]  GI=[0.9 30]  GH=[12.0 115]  GLd=[66 66 9.4]  TcLF=[1.667 2 0 0 0 0 2 2.4 0 0 0 0 1 1]  GId=[66 66 47.6]  TcIF=[1 1 0.25 0.3 0 0 1 1 0.3 0.36 0 0 0 0]  GHd=[66 66 233]  TcHF="[0.01 0.012 0 0 0 0  0.012 0.0144 0 0 0 0 1 1]"  LIM=[.075 .15 .15 .15]  Plot_On=off  MagdB_On=on  FreqRange=logspace(-2,2,500)
  Multiport Switch : MultiPortSwitch
  Sum2 : Sum  Inputs=+-  InputSameDT=on  SaturateOnIntegerOverflow=on  OutDataTypeStr=Inherit: Same as first input
  Stab : Outport  InitialOutput=0  VectorParamsAs1DForOutWhenUnconnected=off
  wires:
  Multi-Band Power System Stabilizer/1 -> Multiport Switch/4
  dw/1 -> Multi-Band Power System Stabilizer/1
  [PSS_select] -> Multiport Switch/1
  Ground1/1 -> Multiport Switch/2
  Pe/1 -> Sum2/2
  Pm/1 -> Sum2/1
  Sum2/1 -> Generic Power System Stabilizer/1
  Generic Power System Stabilizer/1 -> Multiport Switch/3
  Multiport Switch/1 -> Stab/1

== system LoFT_Example3/Onshore grid/Onshore Grid/Subsystem/SG6/Regulators6/Turbine  & Excitation Regulators Mac2/Stabilisateur ==
  Pm : Inport
  Pe : Inport  Port=2
  dw : Inport  Port=3
  Generic Power System Stabilizer : spsGenericPowerSystemStabilizerLib/Generic Power System Stabilizer  Tsensor=15e-3  K=2.5  Twashout=1  Tleadlag1="[0.06  1]"  Tleadlag2="[0  0]"  VSlimits=[-0.15 0.15]  Vinit=0  Plot_On=off  MagdB_On=on  FreqRange=logspace(-2,2,500)
  Ground1 : Ground
  Multi-Band Power System Stabilizer : spsMultiBandPowerSystemStabilizerLib/Multi-Band Power System Stabilizer  OperationMode=Simplified settings  Kg=0.7  GL=[0.2 10]  GI=[0.9 30]  GH=[12.0 115]  GLd=[66 66 9.4]  TcLF=[1.667 2 0 0 0 0 2 2.4 0 0 0 0 1 1]  GId=[66 66 47.6]  TcIF=[1 1 0.25 0.3 0 0 1 1 0.3 0.36 0 0 0 0]  GHd=[66 66 233]  TcHF="[0.01 0.012 0 0 0 0  0.012 0.0144 0 0 0 0 1 1]"  LIM=[.075 .15 .15 .15]  Plot_On=off  MagdB_On=on  FreqRange=logspace(-2,2,500)
  Multiport Switch : MultiPortSwitch
  Sum2 : Sum  Inputs=+-  InputSameDT=on  SaturateOnIntegerOverflow=on  OutDataTypeStr=Inherit: Same as first input
  Stab : Outport  InitialOutput=0  VectorParamsAs1DForOutWhenUnconnected=off
  wires:
  Multi-Band Power System Stabilizer/1 -> Multiport Switch/4
  dw/1 -> Multi-Band Power System Stabilizer/1
  [PSS_select] -> Multiport Switch/1
  Ground1/1 -> Multiport Switch/2
  Pe/1 -> Sum2/2
  Pm/1 -> Sum2/1
  Sum2/1 -> Generic Power System Stabilizer/1
  Generic Power System Stabilizer/1 -> Multiport Switch/3
  Multiport Switch/1 -> Stab/1

== system LoFT_Example3/Onshore grid/Onshore Grid/Subsystem/SG6/Regulators6/Turbine  & Excitation Regulators Mac2/Subsystem ==
  In1 : Inport
  <Rotor speed  wm  (pu)> : Inport  Port=2
  Abs : Abs  SaturateOnIntegerOverflow=off
  Add : Sum  Inputs=+-
  Constant : Constant  Value=0
  Km(1+FH*TR*s)/(1+TR*s) : TransferFcn  Commented=on  Numerator=[0.95*0.25*7.758 0.95]  Denominator=[7.758 1]
  PID Controller : slpidlib/PID Controller  Controller=PID  Form=Parallel  TimeDomain=Discrete-time  UseExternalTs=off  SampleTime=-1  IntegratorMethod=Forward Euler  FilterMethod=Forward Euler  ControllerParametersSource=internal  P=0  I=0.3  UseKiTs=off  D=0  UseExternalDerivativeSource=off  N=100  UseFilter=on  TunerSelectOption=Transfer Function Based (PID Tuner App)  InitialConditionSource=internal  InitialConditionForIntegrator=0  InitialConditionForFilter=0  DifferentiatorICPrevScaledInput=0  ExternalReset=none  TrackingMode=off  Kt=1  LimitOutput=off  SatLimitsSource=internal  UpperSaturationLimit=inf  LowerSaturationLimit=-inf  LinearizeAsGain=on  AntiWindupMode=none  Kb=1  LimitIntegrator=off  UpperIntegratorSaturationLimit=inf  LowerIntegratorSaturationLimit=-inf  POutMin=[]  POutMax=[]  IOutMin=[]  IOutMax=[]  DOutMin=[]  DOutMax=[]  NOutMin=[]  NOutMax=[]  SumOutMin=[]  SumOutMax=[]  SaturationOutMin=[]  SaturationOutMax=[]  PParamMin=[]  PParamMax=[]  IParamMin=[]  IParamMax=[]  DParamMin=[]  DParamMax=[]  NParamMin=[]  NParamMax=[]  KbParamMin=[]  KbParamMax=[]  KtParamMin=[]  KtParamMax=[]  KbOutMin=[]  KbOutMax=[]  KtOutMin=[]  KtOutMax=[]  IntegratorOutMin=[]  IntegratorOutMax=[]  FilterOutMin=[]  FilterOutMax=[]  SumI1OutMin=[]  SumI1OutMax=[]  SumI2OutMin=[]  SumI2OutMax=[]  SumI3OutMin=[]  SumI3OutMax=[]  SumI4OutMin=[]  SumI4OutMax=[]  SumDOutMin=[]  SumDOutMax=[]  DifferentiatorOutMin=[]  DifferentiatorOutMax=[]  FilterDiffOutCoefMin=[]  FilterDiffOutCoefMax=[]  ReciprocalOutMin=[]  ReciprocalOutMax=[]  SumDenOutMin=[]  SumDenOutMax=[]  SumNumOutMin=[]  SumNumOutMax=[]  DivideOutMin=[]  DivideOutMax=[]  UdiffTsProdOutMin=[]  UdiffTsProdOutMax=[]  NTsProdOutMin=[]  NTsProdOutMax=[]  UintegralTsProdOutMin=[]  UintegralTsProdOutMax=[]  UngainTsProdOutMin=[]  UngainTsProdOutMax=[]  ClampingZeroOutDataTypeStr=Inherit: Inherit via back propagation  ClampingZeroOutMin=[]  ClampingZeroOutMax=[]  FilterDenConstantOutDataTypeStr=Inherit: Inherit via back propagation  FilterDenConstantOutMin=[]  FilterDenConstantOutMax=[]  PCopyOutDataTypeStr=Inherit: Inherit via back propagation  PCopyOutMin=[]  PCopyOutMax=[]  NCopyOutDataTypeStr=Inherit: Inherit via back propagation  NCopyOutMin=[]  NCopyOutMax=[]  IntegratorContinuousStateAttributes=''  IntegratorStateMustResolveToSignalObject=off  IntegratorRTWStateStorageClass=Auto  FilterContinuousStateAttributes=''  FilterStateMustResolveToSignalObject=off  FilterRTWStateStorageClass=Auto  ParallelPVariant=InternalParameters  IdealPVariant=Disabled  IVariant=InternalParameters  DVariant=InternalParameters  IntegratorVariant=Discrete  SatVariant=Disabled  AWVariant=Passthrough  PCopyVariant=Disabled  TRVariant=Disabled  FdbkBlocksVariant=Forward  IdealPFdbkVariant=Disabled  SatFdbkVariant=Disabled  DerivativeFilterVariant=ForwardEulerFilter  NVariant=InternalParameters  NCopyVariant=Disabled  FilterICVariant=InternalICsFilter  IntegratorICVariant=InternalICs  ExternalResetVariant=Disabled  TRSumVariant=Passthrough  SumFdbkVariant=Disabled  SumVariant=Sum_PID  TsampFilterVariant=InternalTs  TsampNgainVariant=Passthrough  TsampIntegralVariant=Disabled_SignalSpec  ExternalSaturationOutDataTypeStr=Inherit: Same as second input  DerivativeSourceVariant=ErrorSignal  PreIntVariant=InternalPreInt
  Switch : Switch  Threshold=0.2/50  SaturateOnIntegerOverflow=off  InputSameDT=off
  Out1 : Outport
  wires:
  In1/1 -> Add/1
  Switch/1 -> PID Controller/1
  Add/1 -> Abs/1, Switch/3
  <Rotor speed  wm  (pu)>/1 -> Add/2
  Abs/1 -> Switch/2
  Constant/1 -> Switch/1
  PID Controller/1 -> Out1/1

== system LoFT_Example3/Onshore grid/Onshore Grid/Subsystem/SG8/Regulators8/Turbine  & Excitation Regulators Mac2/Stabilisateur ==
  Pm : Inport
  Pe : Inport  Port=2
  dw : Inport  Port=3
  Generic Power System Stabilizer : spsGenericPowerSystemStabilizerLib/Generic Power System Stabilizer  Tsensor=15e-3  K=2.5  Twashout=1  Tleadlag1="[0.06  1]"  Tleadlag2="[0  0]"  VSlimits=[-0.15 0.15]  Vinit=0  Plot_On=off  MagdB_On=on  FreqRange=logspace(-2,2,500)
  Ground1 : Ground
  Multi-Band Power System Stabilizer : spsMultiBandPowerSystemStabilizerLib/Multi-Band Power System Stabilizer  OperationMode=Simplified settings  Kg=0.7  GL=[0.2 10]  GI=[0.9 30]  GH=[12.0 115]  GLd=[66 66 9.4]  TcLF=[1.667 2 0 0 0 0 2 2.4 0 0 0 0 1 1]  GId=[66 66 47.6]  TcIF=[1 1 0.25 0.3 0 0 1 1 0.3 0.36 0 0 0 0]  GHd=[66 66 233]  TcHF="[0.01 0.012 0 0 0 0  0.012 0.0144 0 0 0 0 1 1]"  LIM=[.075 .15 .15 .15]  Plot_On=off  MagdB_On=on  FreqRange=logspace(-2,2,500)
  Multiport Switch : MultiPortSwitch
  Sum2 : Sum  Inputs=+-  InputSameDT=on  SaturateOnIntegerOverflow=on  OutDataTypeStr=Inherit: Same as first input
  Stab : Outport  InitialOutput=0  VectorParamsAs1DForOutWhenUnconnected=off
  wires:
  Multi-Band Power System Stabilizer/1 -> Multiport Switch/4
  dw/1 -> Multi-Band Power System Stabilizer/1
  [PSS_select] -> Multiport Switch/1
  Ground1/1 -> Multiport Switch/2
  Pe/1 -> Sum2/2
  Pm/1 -> Sum2/1
  Sum2/1 -> Generic Power System Stabilizer/1
  Generic Power System Stabilizer/1 -> Multiport Switch/3
  Multiport Switch/1 -> Stab/1

== system LoFT_Example3/Onshore grid/Onshore Grid/Subsystem/SG8/Regulators8/Turbine  & Excitation Regulators Mac2/Subsystem ==
  In1 : Inport
  <Rotor speed  wm  (pu)> : Inport  Port=2
  Abs : Abs  SaturateOnIntegerOverflow=off
  Add : Sum  Inputs=+-
  Constant : Constant  Value=0
  Km(1+FH*TR*s)/(1+TR*s) : TransferFcn  Commented=on  Numerator=[0.95*0.25*7.758 0.95]  Denominator=[7.758 1]
  PID Controller : slpidlib/PID Controller  Controller=PID  Form=Parallel  TimeDomain=Discrete-time  UseExternalTs=off  SampleTime=-1  IntegratorMethod=Forward Euler  FilterMethod=Forward Euler  ControllerParametersSource=internal  P=0  I=0.3  UseKiTs=off  D=0  UseExternalDerivativeSource=off  N=100  UseFilter=on  TunerSelectOption=Transfer Function Based (PID Tuner App)  InitialConditionSource=internal  InitialConditionForIntegrator=0  InitialConditionForFilter=0  DifferentiatorICPrevScaledInput=0  ExternalReset=none  TrackingMode=off  Kt=1  LimitOutput=off  SatLimitsSource=internal  UpperSaturationLimit=inf  LowerSaturationLimit=-inf  LinearizeAsGain=on  AntiWindupMode=none  Kb=1  LimitIntegrator=off  UpperIntegratorSaturationLimit=inf  LowerIntegratorSaturationLimit=-inf  POutMin=[]  POutMax=[]  IOutMin=[]  IOutMax=[]  DOutMin=[]  DOutMax=[]  NOutMin=[]  NOutMax=[]  SumOutMin=[]  SumOutMax=[]  SaturationOutMin=[]  SaturationOutMax=[]  PParamMin=[]  PParamMax=[]  IParamMin=[]  IParamMax=[]  DParamMin=[]  DParamMax=[]  NParamMin=[]  NParamMax=[]  KbParamMin=[]  KbParamMax=[]  KtParamMin=[]  KtParamMax=[]  KbOutMin=[]  KbOutMax=[]  KtOutMin=[]  KtOutMax=[]  IntegratorOutMin=[]  IntegratorOutMax=[]  FilterOutMin=[]  FilterOutMax=[]  SumI1OutMin=[]  SumI1OutMax=[]  SumI2OutMin=[]  SumI2OutMax=[]  SumI3OutMin=[]  SumI3OutMax=[]  SumI4OutMin=[]  SumI4OutMax=[]  SumDOutMin=[]  SumDOutMax=[]  DifferentiatorOutMin=[]  DifferentiatorOutMax=[]  FilterDiffOutCoefMin=[]  FilterDiffOutCoefMax=[]  ReciprocalOutMin=[]  ReciprocalOutMax=[]  SumDenOutMin=[]  SumDenOutMax=[]  SumNumOutMin=[]  SumNumOutMax=[]  DivideOutMin=[]  DivideOutMax=[]  UdiffTsProdOutMin=[]  UdiffTsProdOutMax=[]  NTsProdOutMin=[]  NTsProdOutMax=[]  UintegralTsProdOutMin=[]  UintegralTsProdOutMax=[]  UngainTsProdOutMin=[]  UngainTsProdOutMax=[]  ClampingZeroOutDataTypeStr=Inherit: Inherit via back propagation  ClampingZeroOutMin=[]  ClampingZeroOutMax=[]  FilterDenConstantOutDataTypeStr=Inherit: Inherit via back propagation  FilterDenConstantOutMin=[]  FilterDenConstantOutMax=[]  PCopyOutDataTypeStr=Inherit: Inherit via back propagation  PCopyOutMin=[]  PCopyOutMax=[]  NCopyOutDataTypeStr=Inherit: Inherit via back propagation  NCopyOutMin=[]  NCopyOutMax=[]  IntegratorContinuousStateAttributes=''  IntegratorStateMustResolveToSignalObject=off  IntegratorRTWStateStorageClass=Auto  FilterContinuousStateAttributes=''  FilterStateMustResolveToSignalObject=off  FilterRTWStateStorageClass=Auto  ParallelPVariant=InternalParameters  IdealPVariant=Disabled  IVariant=InternalParameters  DVariant=InternalParameters  IntegratorVariant=Discrete  SatVariant=Disabled  AWVariant=Passthrough  PCopyVariant=Disabled  TRVariant=Disabled  FdbkBlocksVariant=Forward  IdealPFdbkVariant=Disabled  SatFdbkVariant=Disabled  DerivativeFilterVariant=ForwardEulerFilter  NVariant=InternalParameters  NCopyVariant=Disabled  FilterICVariant=InternalICsFilter  IntegratorICVariant=InternalICs  ExternalResetVariant=Disabled  TRSumVariant=Passthrough  SumFdbkVariant=Disabled  SumVariant=Sum_PID  TsampFilterVariant=InternalTs  TsampNgainVariant=Passthrough  TsampIntegralVariant=Disabled_SignalSpec  ExternalSaturationOutDataTypeStr=Inherit: Same as second input  DerivativeSourceVariant=ErrorSignal  PreIntVariant=InternalPreInt
  Switch : Switch  Threshold=0.2/50  SaturateOnIntegerOverflow=off  InputSameDT=off
  Out1 : Outport
  wires:
  In1/1 -> Add/1
  Switch/1 -> PID Controller/1
  Add/1 -> Abs/1, Switch/3
  <Rotor speed  wm  (pu)>/1 -> Add/2
  Abs/1 -> Switch/2
  Constant/1 -> Switch/1
  PID Controller/1 -> Out1/1
